simulink model "button_to_led2"  (R2017a)
settings: Solver=FixedStepDiscrete  StartTime=0.0  StopTime=500000  FixedStep=1  RelTol=1e-3
libraries: hdlsllib x2, simulink x1
settings Model: Creator=Patrick  LastModifiedBy=Patrick
settings SFSimCC: SimUseLocalCustomCode=on
settings RTWCC: RTWUseLocalCustomCode=on

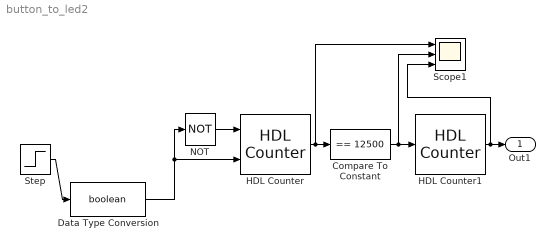
== system button_to_led2 ==
  Compare To Constant : simulink/Logic and Bit Operations/Compare To Constant  relop===  const=12500  OutDataTypeStr=boolean
  Data Type Conversion : DataTypeConversion  OutDataTypeStr=boolean
  HDL Counter : hdlsllib/HDL Operations/HDL Counter  CountType=Count limited  CountInit=0  CountStep=1  CountMax=50000  CountFromType=Initial value  CountFrom=0  CountResetPort=on  CountLoadPort=off  CountEnbPort=on  CountDirPort=off  CountDataType=Unsigned  CountWordLen=50  CountFracLen=0  CountSampTime=1
      settings: SourceProductName=HDL Coder  SourceProductBaseCode=HD
  HDL Counter1 : hdlsllib/HDL Operations/HDL Counter  CountType=Free running  CountInit=0  CountStep=1  CountMax=25  CountFromType=Initial value  CountFrom=0  CountResetPort=off  CountLoadPort=off  CountEnbPort=on  CountDirPort=off  CountDataType=Unsigned  CountWordLen=1  CountFracLen=0  CountSampTime=1
      settings: SourceProductName=HDL Coder  SourceProductBaseCode=HD
  NOT : Logic  Operator=NOT  IconShape=distinctive  AllPortsSameDT=off  OutDataTypeStr=boolean
  Scope1 : Scope  NumInputPorts=3
  Step : Step  Time=25000  SampleTime=1
  Out1 : Outport  SampleTime=1
  wires:
  HDL Counter/1 -> Scope1/1, Compare To Constant/1
  Compare To Constant/1 -> Scope1/2, HDL Counter1/1
  Step/1 -> Data Type Conversion/1
  NOT/1 -> HDL Counter/1
  HDL Counter1/1 -> Scope1/3, Out1/1
  Data Type Conversion/1 -> NOT/1, HDL Counter/2
